simulink subsystem "RackAndPinion"  (R2023a)
settings: Solver=VariableStepAuto  StartTime=0.0  StopTime=10.0  RelTol=1e-3
values from neighbouring files (symbols this model uses):
  i_rail = 20 * 1000    (= 20000)    [constants.m]
  J_rail = 5    [constants.m]
  k_visco = 0.05    [constants.m]
  m_rail = 0.5    [constants.m]
settings Model: Creator=ПК  LastModifiedBy=ycheb

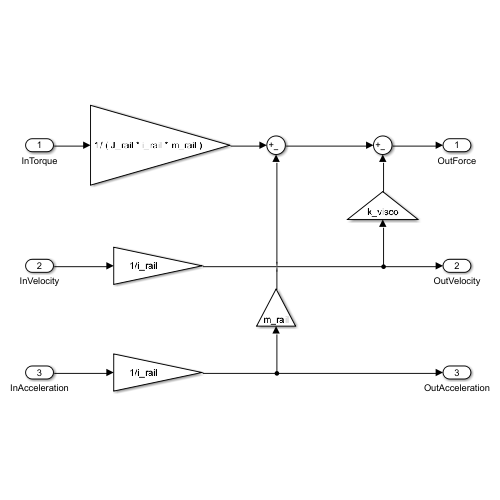
[thumbnail: Simulink's stored preview of the top-level diagram]
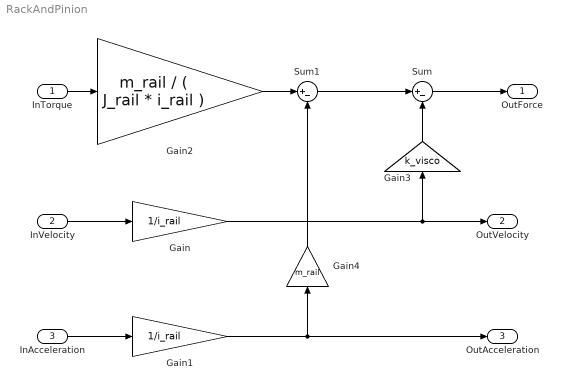
== system RackAndPinion ==
  InTorque : Inport
  InVelocity : Inport  Port=2
  InAcceleration : Inport  Port=3
  Gain : Gain  Gain=1/i_rail
  Gain1 : Gain  Gain=1/i_rail
  Gain2 : Gain  Gain=m_rail / ( J_rail * i_rail )
  Gain3 : Gain  Gain=k_visco
  Gain4 : Gain  Gain=m_rail
  Sum : Sum  Inputs=|+-
  Sum1 : Sum  Inputs=|+-
  OutForce : Outport
  OutVelocity : Outport  Port=2
  OutAcceleration : Outport  Port=3
  wires:
  InVelocity/1 -> Gain/1
  Gain/1 -> OutVelocity/1, Gain3/1
  InAcceleration/1 -> Gain1/1
  Gain1/1 -> Gain4/1, OutAcceleration/1
  InTorque/1 -> Gain2/1
  Gain3/1 -> Sum/2
  Gain2/1 -> Sum1/1
  Sum1/1 -> Sum/1
  Gain4/1 -> Sum1/2
  Sum/1 -> OutForce/1
